simulink model "vrmaglev_sys"  (R2021b)
settings: Solver=VariableStepAuto  StartTime=0.0  StopTime=5  RelTol=1e-3
model workspace (MAT data in the model file):
  M = Simulink.Parameter
  M.DataType = 'auto'
  M.Complexity = 'real'
  M.Dimensions = [0 0]
values from neighbouring files (symbols this model uses):
  c = 0.3    [Section9_Initialization.m]
  fv = 0.04    [Section9_Initialization.m]
  L = 0.2    [Section9_Initialization.m]
  R = 50    [Section9_Initialization.m]
libraries: vrlib x2, slpidlib x1
settings Model: Creator=USER  LastModifiedBy=odeut

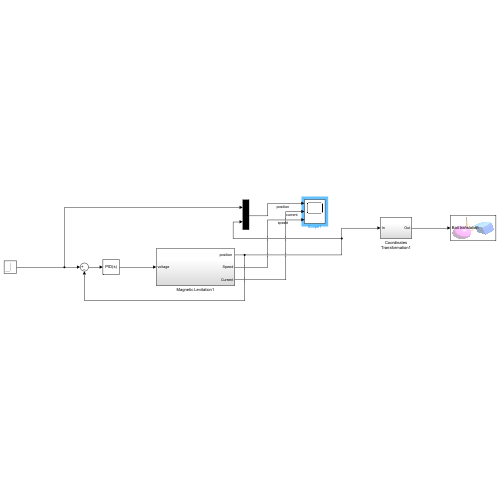
[thumbnail: Simulink's stored preview of the top-level diagram]
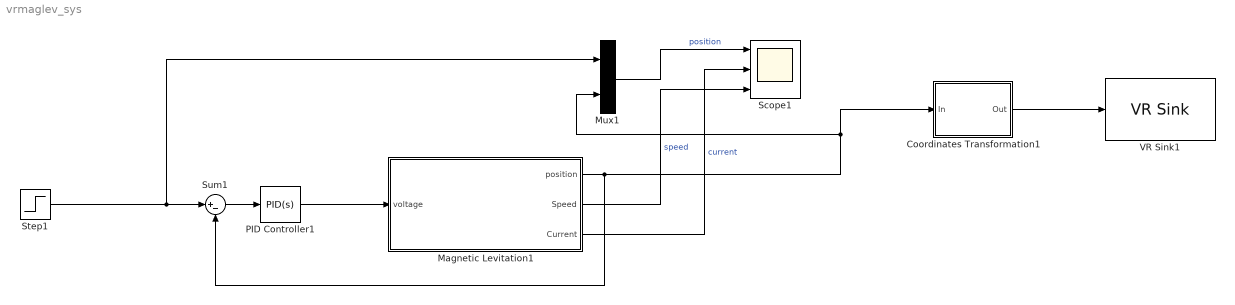
== system vrmaglev_sys ==
  Coordinates Transformation1 : Subsystem
  Magnetic Levitation1 : Subsystem
  Mux1 : Mux  Inputs=2
  PID Controller1 : slpidlib/PID Controller  Controller=PID  Form=Parallel  TimeDomain=Continuous-time  UseExternalTs=off  SampleTime=-1  IntegratorMethod=Forward Euler  FilterMethod=Forward Euler  ControllerParametersSource=internal  P=1278.8604861075  I=3736.57027457271  D=101.778616391159  UseFilter=on  N=5547.15345605962  TunerSelectOption=Transfer Function Based (PID Tuner App)  InitialConditionSource=internal  InitialConditionForIntegrator=0  InitialConditionForFilter=0  DifferentiatorICPrevScaledInput=0  ExternalReset=none  TrackingMode=off  Kt=1  LimitOutput=off  SatLimitsSource=internal  UpperSaturationLimit=inf  LowerSaturationLimit=-inf  LinearizeAsGain=on  AntiWindupMode=none  Kb=1  POutMin=[]  POutMax=[]  IOutMin=[]  IOutMax=[]  DOutMin=[]  DOutMax=[]  NOutMin=[]  NOutMax=[]  SumOutMin=[]  SumOutMax=[]  SaturationOutMin=[]  SaturationOutMax=[]  PParamMin=[]  PParamMax=[]  IParamMin=[]  IParamMax=[]  DParamMin=[]  DParamMax=[]  NParamMin=[]  NParamMax=[]  KbParamMin=[]  KbParamMax=[]  KtParamMin=[]  KtParamMax=[]  KbOutMin=[]  KbOutMax=[]  KtOutMin=[]  KtOutMax=[]  IntegratorOutMin=[]  IntegratorOutMax=[]  FilterOutMin=[]  FilterOutMax=[]  SumI1OutMin=[]  SumI1OutMax=[]  SumI2OutMin=[]  SumI2OutMax=[]  SumI3OutMin=[]  SumI3OutMax=[]  SumI4OutMin=[]  SumI4OutMax=[]  SumDOutMin=[]  SumDOutMax=[]  DifferentiatorOutMin=[]  DifferentiatorOutMax=[]  FilterDiffOutCoefMin=[]  FilterDiffOutCoefMax=[]  ReciprocalOutMin=[]  ReciprocalOutMax=[]  SumDenOutMin=[]  SumDenOutMax=[]  SumNumOutMin=[]  SumNumOutMax=[]  DivideOutMin=[]  DivideOutMax=[]  UdiffTsProdOutMin=[]  UdiffTsProdOutMax=[]  NTsProdOutMin=[]  NTsProdOutMax=[]  UintegralTsProdOutMin=[]  UintegralTsProdOutMax=[]  UngainTsProdOutMin=[]  UngainTsProdOutMax=[]  IntegratorContinuousStateAttributes=''  IntegratorStateMustResolveToSignalObject=off  IntegratorRTWStateStorageClass=Auto  FilterContinuousStateAttributes=''  FilterStateMustResolveToSignalObject=off  FilterRTWStateStorageClass=Auto  ParallelPVariant=InternalParameters  IdealPVariant=Disabled  IVariant=InternalParameters  DVariant=InternalParameters  IntegratorVariant=Continuous  SatVariant=Disabled  AWVariant=Passthrough  PCopyVariant=Disabled  TRVariant=Disabled  FdbkBlocksVariant=Forward  IdealPFdbkVariant=Disabled  SatFdbkVariant=Disabled  DerivativeFilterVariant=ContFilter  NVariant=InternalParameters  NCopyVariant=Disabled  FilterICVariant=InternalICsFilter  IntegratorICVariant=InternalICs  ExternalResetVariant=Disabled  TRSumVariant=Passthrough  SumFdbkVariant=Disabled  SumVariant=Sum_PID  TsampFilterVariant=InternalTs  TsampNgainVariant=Passthrough  TsampIntegralVariant=Passthrough  ExternalSaturationOutDataTypeStr=Inherit: Same as second input
  Scope1 : Scope  NumInputPorts=3
  Step1 : Step  Time=0  After=0.06  SampleTime=0
  Sum1 : Sum  Inputs=|+-
  VR Sink1 : vrlib/VR Sink  InstantiateOnLoad=on  SampleTime=0.02  ViewEnable=on  RemoteChange=off  RemoteView=off  FieldsWritten=Ball.translation.3.1.1.double  WorldFileName=maglev.wrl  WorldDescription=VR Magnetic Levitation Model  AutoView=on  VideoDimensions=[]  AllowVariableSize=off  FigureProperties="{'Position', 'Name', 'Viewpoint', 'CameraBound', 'CameraDirection', 'CameraPosition', 'CameraUpVector', 'ZoomFactor', 'Antialiasing', 'Headlight', 'Lighting', 'NavPanel', 'Sound', 'StatusBar', 'Stereo3D', 'Stereo3DCameraOffset', 'Stereo3DHIT', 'ToolBar', 'Textures', 'Transparency', 'Triad', 'Wireframe', 'NavZones', 'NavMode', 'NavSpeed', 'CaptureFileFormat', 'CaptureFileName', 'Record2DCompressMethod', 'Record2DCompressQuality', 'Record2D', 'Record2DFileName', 'Record2DFPS'; [5.0000000000000000e+00   9.2000000000000000e+01   5.7600000000000000e+02   3.5000000000000000e+02], 'VR Magnetic Levitation Model', 'Camera 1', 'on', [0.0000000000000000e+00   0.0000000000000000e+00  -1.0000000000000000e+00], [0.0000000000000000e+00   0.0000000000000000e+00   0.0000000000000000e+00], [0.0000000000000000e+00   1.0000000000000000e+00   0.0000000000000000e+00], [1.0000000000000000e+00], 'on', 'off', 'on', 'halfbar', 'on', 'on', 'off', [1.0000000149011612e-01], [0.0000000000000000e+00], 'on', 'on', 'on', 'none', 'off', 'off', 'examine', 'normal', 'tif', '%f_anim_%n.tif', 'auto', [7.5000000000000000e+01], 'off', '%f_anim_%n.avi', 'auto'}"
      settings: SourceProductBaseCode=VR
  wires:
  Coordinates Transformation1/1(Out) -> VR Sink1/1
  Mux1/1 -> Scope1/1  "position"
  Magnetic Levitation1/1("position ") -> Coordinates Transformation1/1(In), Mux1/2, Sum1/2
  Step1/1 -> Sum1/1, Mux1/1
  PID Controller1/1 -> Magnetic Levitation1/1(voltage)
  Sum1/1 -> PID Controller1/1
  Magnetic Levitation1/2(Speed) -> Scope1/3  "speed"
  Magnetic Levitation1/3(Current) -> Scope1/2  "current"

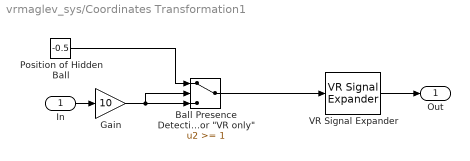
== system vrmaglev_sys/Coordinates Transformation1 ==
  In : Inport
  "Ball Presence Detection Value > Threshold = Ball Not Present 1 for \"VR only\"" : Switch  Threshold=1  InputSameDT=on
  Gain : Gain  Gain=10
  Position of Hidden Ball : Constant  Value=-0.5
  VR Signal Expander : vrlib/VR Signal Expander  outwidth=3  outidx=[2]
      settings: SourceProductBaseCode=VR
  Out : Outport  VectorParamsAs1DForOutWhenUnconnected=off
  wires:
  Position of Hidden Ball/1 -> "Ball Presence Detection Value > Threshold = Ball Not Present 1 for \"VR only\""/1
  In/1 -> Gain/1
  "Ball Presence Detection Value > Threshold = Ball Not Present 1 for \"VR only\""/1 -> VR Signal Expander/1
  VR Signal Expander/1 -> Out/1
  Gain/1 -> "Ball Presence Detection Value > Threshold = Ball Not Present 1 for \"VR only\""/3, "Ball Presence Detection Value > Threshold = Ball Not Present 1 for \"VR only\""/2

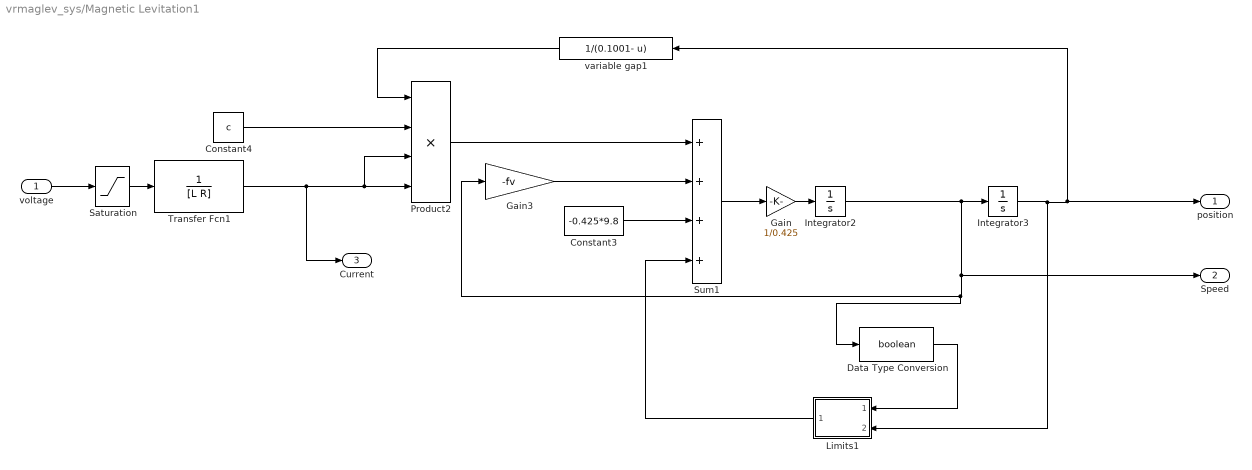
== system vrmaglev_sys/Magnetic Levitation1 ==
  voltage : Inport
  Constant3 : Constant  Value=-0.425*9.8
  Constant4 : Constant  Value=c
  Data Type Conversion : DataTypeConversion  OutDataTypeStr=boolean
  Gain : Gain  Gain=1/0.425
  Gain3 : Gain  Gain=-fv
  Integrator2 : Integrator  LowerSaturationLimit=0
  Integrator3 : Integrator  InitialCondition=0.0001  LimitOutput=on  UpperSaturationLimit=0.1  LowerSaturationLimit=0
  Limits1 : Subsystem
      mask Display: disp('LIMIT')
  Product2 : Product  Inputs=4
  Saturation : Saturate  UpperLimit=200  LowerLimit=0  ZeroCross=off
  Sum1 : Sum  Inputs=++++
  Transfer Fcn1 : TransferFcn  Denominator=[L R]
  variable gap1 : Fcn  Expr=1/(0.1001- u)
  "position " : Outport  VectorParamsAs1DForOutWhenUnconnected=off
  Speed : Outport  Port=2  VectorParamsAs1DForOutWhenUnconnected=off
  Current : Outport  Port=3  VectorParamsAs1DForOutWhenUnconnected=off
  wires:
  Constant3/1 -> Sum1/3
  Transfer Fcn1/1 -> Current/1, Product2/3, Product2/4
  Sum1/1 -> Gain/1
  Saturation/1 -> Transfer Fcn1/1
  Integrator2/1 -> Speed/1, Data Type Conversion/1, Gain3/1, Integrator3/1
  Limits1/1(force) -> Sum1/4
  Constant4/1 -> Product2/2
  Product2/1 -> Sum1/1
  Gain/1 -> Integrator2/1
  Gain3/1 -> Sum1/2
  variable gap1/1 -> Product2/1
  voltage/1 -> Saturation/1
  Integrator3/1 -> Limits1/2(position), "position "/1, variable gap1/1
  Data Type Conversion/1 -> Limits1/1(velocity)

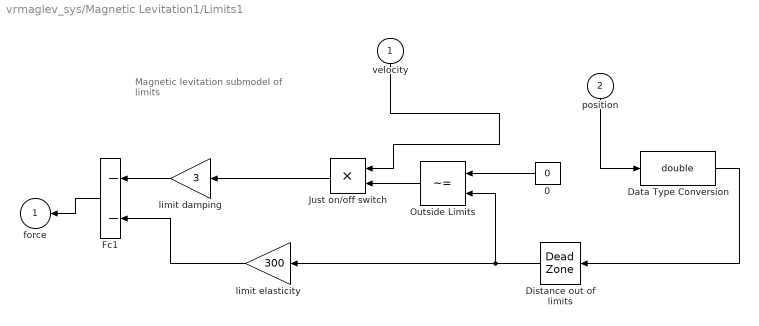
== system vrmaglev_sys/Magnetic Levitation1/Limits1 ==
  note: Magnetic levitation
      | submodel of limits
  velocity : Inport
  position : Inport  Port=2
  0 : Constant  Value=0
  Data Type Conversion : DataTypeConversion  OutDataTypeStr=double
  Distance out of limits : DeadZone  LowerValue=0.0002  UpperValue=0.0998  ZeroCross=off  SaturateOnIntegerOverflow=on
  Fc1 : Sum  Inputs=--  InputSameDT=on  SaturateOnIntegerOverflow=on  OutDataTypeStr=Inherit: Same as first input
  "Just on/off switch " : Product  InputSameDT=on  OutDataTypeStr=double  SaturateOnIntegerOverflow=on
  Outside Limits : RelationalOperator  Operator=~=  RndMeth=Nearest  InputSameDT=on
  limit damping : Gain  Gain=3  OutDataTypeStr=double  SaturateOnIntegerOverflow=on  ParamDataTypeStr=Inherit: Same as input
  limit elasticity : Gain  Gain=300  OutDataTypeStr=double  SaturateOnIntegerOverflow=on  ParamDataTypeStr=Inherit: Same as input
  force : Outport  VectorParamsAs1DForOutWhenUnconnected=off
  wires:
  Distance out of limits/1 -> Outside Limits/2, limit elasticity/1
  limit damping/1 -> Fc1/1
  limit elasticity/1 -> Fc1/2
  Outside Limits/1 -> "Just on/off switch "/2
  0/1 -> Outside Limits/1
  Fc1/1 -> force/1
  position/1 -> Data Type Conversion/1
  Data Type Conversion/1 -> Distance out of limits/1
  velocity/1 -> "Just on/off switch "/1
  "Just on/off switch "/1 -> limit damping/1
